simulink model "sampleModel1907"  (R2023a)
settings: Solver=VariableStepAuto  StartTime=0.0  StopTime=10.0  RelTol=1e-3
libraries: hdlsllib x5, simulink x4
settings Model: Creator=user1  LastModifiedBy=user1

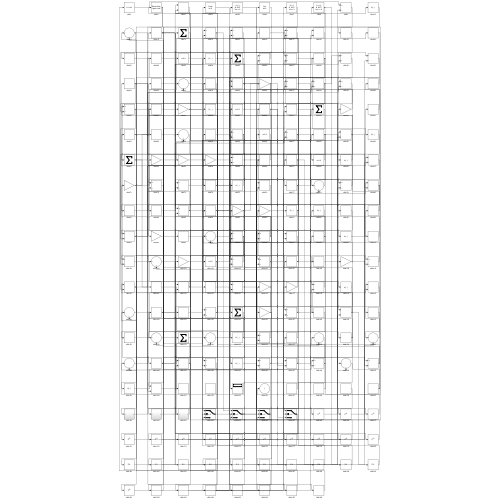
[thumbnail: Simulink's stored preview of the top-level diagram]
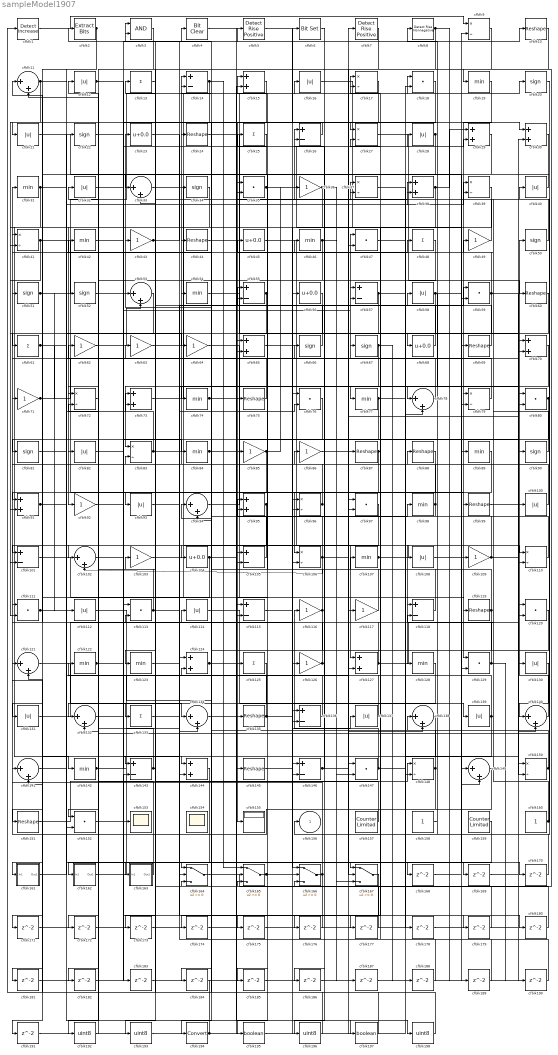
== system sampleModel1907 ==
  cfblk1 : simulink/Logic and Bit Operations/Detect Increase  vinit=0.0  OutDataTypeStr=boolean
      settings: LibrarySourceBlock=|
      | hdlsllib/Logic and Bit
      | Operations/Detect
      | Increase
  cfblk{10,24,44,60,69,75,87..88,99,119,135,145,151} (13 alike) : Reshape
  cfblk{12,16,21,28,32,40,58,82,93,100,108,112,114,130..131,137,139} (17 alike) : Abs  SaturateOnIntegerOverflow=off
  cfblk{14,26,55,57,101,105,115,118,136,143,146} (11 alike) : Sum  Inputs=+-
  cfblk{11,33,53,78,94,102,121,132,134,138,140..141,149} (13 alike) : Sum  Inputs=|++
  cfblk{36,43,49,62..64,71,85..86,92,103,109,116..117,126} (15 alike) : Gain
  cfblk{23,45,56,68,104} (5 alike) : Bias  Bias=0.0  SaturateOnIntegerOverflow=off
  cfblk{9,17,27,37,39,41,72,79,83,96,106,110,148,150} (14 alike) : Product  Inputs=*/  RndMeth=Zero  SaturateOnIntegerOverflow=on
  cfblk{19,31,42,46,54,74,77,84,89,98,107,122..123,128,142} (15 alike) : MinMax
  cfblk{18,35,47,59,76,80,97,111,113,120,129,147,152} (13 alike) : DotProduct  OutDataTypeStr=Inherit: Inherit via internal rule
  cfblk{15,29..30,38,65,70,73,91,95,124,127,144} (12 alike) : Sum
  cfblk{13,25,48,61,125,133} (6 alike) : Sum  Inputs=+
  cfblk153 : Scope
  cfblk154 : Scope
      settings: Floating=on
  cfblk155 : Display
  cfblk157 : hdlsllib/Sources/Counter Limited  uplimit=7  tsamp=-1
  cfblk158 : Constant  SampleTime=-1
  cfblk159 : hdlsllib/Sources/Counter Limited  uplimit=7  tsamp=-1
  cfblk160 : Constant  SampleTime=-1
  cfblk161 : Subsystem
      settings: LibrarySourceBlock=|
      | hdlsllib/Ports &
      | Subsystems/Subsystem
  cfblk162 : Subsystem
      settings: LibrarySourceBlock=|
      | hdlsllib/Ports &
      | Subsystems/Subsystem
  cfblk163 : Subsystem
      settings: LibrarySourceBlock=|
      | hdlsllib/Ports &
      | Subsystems/Subsystem
  cfblk{164..167} (4 alike) : Switch  SaturateOnIntegerOverflow=off  InputSameDT=off
  cfblk{168..191} (24 alike) : Delay  SampleTime=1
  cfblk{192..193,196,198} (4 alike) : DataTypeConversion  OutDataTypeStr=uint8  SaturateOnIntegerOverflow=off  RndMeth=Floor
  cfblk194 : DataTypeConversion  SaturateOnIntegerOverflow=off  RndMeth=Floor
  cfblk195 : DataTypeConversion  OutDataTypeStr=boolean  SaturateOnIntegerOverflow=off  RndMeth=Floor
  cfblk197 : DataTypeConversion  OutDataTypeStr=boolean  SaturateOnIntegerOverflow=off  RndMeth=Floor
  cfblk2 : simulink/Logic and Bit Operations/Extract Bits  bitsToExtract=Upper half  numBits=8  bitIdxRange=[0 7]  outScalingMode=Preserve fixed-point scaling
      settings: LibrarySourceBlock=|
      | hdlsllib/Logic and Bit
      | Operations/Extract Bits
  cfblk{20,22,34,50..52,66..67,81,90} (10 alike) : Signum
  cfblk3 : Logic  AllPortsSameDT=off  OutDataTypeStr=boolean
  cfblk4 : simulink/Logic and Bit Operations/Bit Clear  iBit=0
      settings: LibrarySourceBlock=|
      | hdlsllib/Logic and Bit
      | Operations/Bit Clear
  cfblk5 : hdlsllib/Logic and Bit Operations/Detect Rise Positive  vinit=0  OutDataTypeStr=boolean
  cfblk6 : simulink/Logic and Bit Operations/Bit Set  iBit=0
      settings: LibrarySourceBlock=|
      | hdlsllib/Logic and Bit
      | Operations/Bit Set
  cfblk7 : hdlsllib/Logic and Bit Operations/Detect Rise Positive  vinit=0  OutDataTypeStr=boolean
  cfblk8 : hdlsllib/Logic and Bit Operations/Detect Rise Nonnegative  vinit=0  OutDataTypeStr=boolean
  cfblk156 : Outport  VectorParamsAs1DForOutWhenUnconnected=off
  wires:
  cfblk18/1 -> cfblk155/1
  cfblk50/1 -> cfblk26/1
  cfblk66/1 -> cfblk13/1
  cfblk121/1 -> cfblk134/1
  cfblk140/1 -> cfblk50/1
  cfblk31/1 -> cfblk142/1, cfblk163/1(In1), cfblk197/1
  cfblk19/1 -> cfblk129/1
  cfblk34/1 -> cfblk92/1
  cfblk130/1 -> cfblk140/1
  cfblk112/1 -> cfblk144/1
  cfblk64/1 -> cfblk119/1
  cfblk61/1 -> cfblk112/1, cfblk38/2
  cfblk149/1 -> cfblk31/1
  cfblk51/1 -> cfblk16/1, cfblk39/2
  cfblk52/1 -> cfblk23/1
  cfblk84/1 -> cfblk99/1, cfblk58/1, cfblk37/2
  cfblk89/1 -> cfblk93/1
  cfblk45/1 -> cfblk79/1
  cfblk127/1 -> cfblk120/1, cfblk94/2
  cfblk87/1 -> cfblk106/1, cfblk37/1
  cfblk101/1 -> cfblk128/1
  cfblk143/1 -> cfblk111/1, cfblk173/1
  cfblk41/1 -> cfblk105/1, cfblk111/2
  cfblk114/1 -> cfblk139/1
  cfblk105/1 -> cfblk53/1
  cfblk98/1 -> cfblk14/1, cfblk95/2
  cfblk139/1 -> cfblk49/1, cfblk26/2, cfblk141/2
  cfblk20/1 -> cfblk156/1
  cfblk147/1 -> cfblk116/1, cfblk150/2
  cfblk74/1 -> cfblk127/1, cfblk14/2, cfblk110/2
  cfblk160/1 -> cfblk114/1, cfblk40/1
  cfblk72/1 -> cfblk102/1
  cfblk131/1 -> cfblk56/1
  cfblk103/1 -> cfblk149/1
  cfblk94/1 -> cfblk20/1
  cfblk26/1 -> cfblk21/1
  cfblk135/1 -> cfblk62/1, cfblk67/1
  cfblk44/1 -> cfblk68/1
  cfblk67/1 -> cfblk75/1, cfblk188/1
  cfblk136/1 -> cfblk12/1
  cfblk21/1 -> cfblk69/1
  cfblk53/1 -> cfblk131/1
  cfblk106/1 -> cfblk102/2, cfblk80/1, cfblk2/1
  cfblk33/1 -> cfblk166/1
  cfblk70/1 -> cfblk83/1
  cfblk77/1 -> cfblk82/1, cfblk80/2
  cfblk58/1 -> cfblk89/1, cfblk78/1, cfblk148/2
  cfblk79/1 -> cfblk51/1
  cfblk138/1 -> cfblk162/1(In1)
  cfblk40/1 -> cfblk33/1
  cfblk78/1 -> cfblk47/1
  cfblk73/1 -> cfblk18/1
  cfblk158/1 -> cfblk88/1
  cfblk91/1 -> cfblk73/1, cfblk48/1
  cfblk133/1 -> cfblk134/2
  cfblk62/1 -> cfblk53/2
  cfblk92/1 -> cfblk113/1
  cfblk83/1 -> cfblk106/2, cfblk73/2
  cfblk115/1 -> cfblk57/1
  cfblk157/1 -> cfblk103/1
  cfblk13/1 -> cfblk123/1
  cfblk95/1 -> cfblk121/2, cfblk193/1
  cfblk75/1 -> cfblk54/1
  cfblk150/1 -> cfblk138/1, cfblk72/2
  cfblk162/1(Out1) -> cfblk47/2
  cfblk57/1 -> cfblk145/1, cfblk78/2
  cfblk109/1 -> cfblk130/1, cfblk15/1
  cfblk148/1 -> cfblk44/1, cfblk177/1
  cfblk63/1 -> cfblk136/1
  cfblk71/1 -> cfblk70/1, cfblk52/1
  cfblk152/1 -> cfblk148/1
  cfblk119/1 -> cfblk107/1, cfblk185/1
  cfblk32/1 -> cfblk153/1
  cfblk86/1 -> cfblk87/1
  cfblk88/1 -> cfblk133/1
  cfblk17/1 -> cfblk74/1
  cfblk120/1 -> cfblk164/1
  cfblk65/1 -> cfblk118/1
  cfblk28/1 -> cfblk91/1, cfblk135/1
  cfblk80/1 -> cfblk115/1, cfblk171/1
  cfblk113/1 -> cfblk59/1, cfblk11/2
  cfblk25/1 -> cfblk115/2
  cfblk107/1 -> cfblk110/1, cfblk27/2
  cfblk12/1 -> cfblk84/1, cfblk152/1, cfblk179/1, cfblk180/1
  cfblk46/1 -> cfblk147/2, cfblk167/3, cfblk172/1
  cfblk116/1 -> cfblk95/1, cfblk165/2
  cfblk146/1 -> cfblk46/1, cfblk138/2
  cfblk142/1 -> cfblk76/2, cfblk29/2
  cfblk29/1 -> cfblk125/1
  cfblk43/1 -> cfblk10/1, cfblk176/1
  cfblk99/1 -> cfblk90/1
  cfblk35/1 -> cfblk109/1, cfblk28/1
  cfblk85/1 -> cfblk161/1(In1), cfblk36/1
  cfblk8/1 -> cfblk33/2, cfblk189/1
  cfblk164/1 -> cfblk19/1
  cfblk110/1 -> cfblk41/1
  cfblk47/1 -> cfblk108/1
  cfblk36/1 -> cfblk91/2, cfblk61/1, cfblk187/1
  cfblk24/1 -> cfblk126/1
  cfblk100/1 -> cfblk17/1
  cfblk55/1 -> cfblk132/1, cfblk184/1
  cfblk82/1 -> cfblk24/1
  cfblk118/1 -> cfblk34/1
  cfblk15/1 -> cfblk104/1
  cfblk151/1 -> cfblk117/1
  cfblk124/1 -> cfblk98/1, cfblk94/1
  cfblk48/1 -> cfblk146/2
  cfblk23/1 -> cfblk77/1
  cfblk90/1 -> cfblk39/1
  cfblk111/1 -> cfblk63/1, cfblk181/1
  cfblk16/1 -> cfblk149/2
  cfblk39/1 -> cfblk167/1
  cfblk5/1 -> cfblk27/1
  cfblk1/1 -> cfblk9/1
  cfblk68/1 -> cfblk43/1
  cfblk159/1 -> cfblk194/1
  cfblk54/1 -> cfblk150/1
  cfblk2/1 -> cfblk101/1, cfblk152/2
  cfblk166/1 -> cfblk141/1, cfblk165/3
  cfblk76/1 -> cfblk96/2
  cfblk42/1 -> cfblk5/1
  cfblk9/1 -> cfblk65/2
  cfblk125/1 -> cfblk132/2
  cfblk96/1 -> cfblk71/1, cfblk3/2
  cfblk104/1 -> cfblk85/1, cfblk151/1
  cfblk27/1 -> cfblk60/1
  cfblk30/1 -> cfblk35/2
  cfblk137/1 -> cfblk122/1
  cfblk161/1(Out1) -> cfblk66/1
  cfblk117/1 -> cfblk86/1
  cfblk56/1 -> cfblk143/1
  cfblk129/1 -> cfblk8/1, cfblk190/1
  cfblk122/1 -> cfblk57/2, cfblk144/2
  cfblk141/1 -> cfblk124/2
  cfblk123/1 -> cfblk55/1
  cfblk163/1(Out1) -> cfblk42/1
  cfblk81/1 -> cfblk22/1
  cfblk49/1 -> cfblk3/1
  cfblk38/1 -> cfblk136/2, cfblk29/1, cfblk55/2
  cfblk10/1 -> cfblk167/2
  cfblk3/1 -> cfblk72/1
  cfblk165/1 -> cfblk137/1, cfblk38/1
  cfblk14/1 -> cfblk81/1, cfblk165/1
  cfblk22/1 -> cfblk30/1
  cfblk69/1 -> cfblk45/1
  cfblk60/1 -> cfblk101/2
  cfblk126/1 -> cfblk11/1, cfblk186/1
  cfblk59/1 -> cfblk100/1, cfblk97/2, cfblk25/1
  cfblk11/1 -> cfblk64/1, cfblk41/2
  cfblk134/1 -> cfblk105/2
  cfblk102/1 -> cfblk168/1
  cfblk168/1 -> cfblk59/2
  cfblk145/1 -> cfblk169/1
  cfblk169/1 -> cfblk140/2
  cfblk108/1 -> cfblk170/1
  cfblk170/1 -> cfblk118/2
  cfblk171/1 -> cfblk120/2
  cfblk172/1 -> cfblk76/1
  cfblk173/1 -> cfblk129/2
  cfblk167/1 -> cfblk174/1
  cfblk174/1 -> cfblk96/1
  cfblk93/1 -> cfblk175/1
  cfblk175/1 -> cfblk147/1
  cfblk176/1 -> cfblk164/2
  cfblk177/1 -> cfblk166/2
  cfblk37/1 -> cfblk178/1
  cfblk178/1 -> cfblk70/2
  cfblk179/1 -> cfblk83/2
  cfblk180/1 -> cfblk166/3
  cfblk181/1 -> cfblk143/2
  cfblk144/1 -> cfblk182/1
  cfblk182/1 -> cfblk35/1
  cfblk132/1 -> cfblk183/1
  cfblk183/1 -> cfblk127/2
  cfblk184/1 -> cfblk1/1
  cfblk185/1 -> cfblk79/2
  cfblk186/1 -> cfblk30/2
  cfblk187/1 -> cfblk9/2
  cfblk188/1 -> cfblk124/1
  cfblk189/1 -> cfblk17/2
  cfblk190/1 -> cfblk164/3
  cfblk97/1 -> cfblk191/1
  cfblk191/1 -> cfblk65/1
  cfblk7/1 -> cfblk192/1
  cfblk192/1 -> cfblk32/1
  cfblk193/1 -> cfblk7/1
  cfblk194/1 -> cfblk15/2, cfblk113/2, cfblk18/2, cfblk97/1
  cfblk128/1 -> cfblk195/1
  cfblk195/1 -> cfblk6/1
  cfblk6/1 -> cfblk196/1
  cfblk196/1 -> cfblk146/1
  cfblk197/1 -> cfblk4/1
  cfblk4/1 -> cfblk198/1
  cfblk198/1 -> cfblk121/1

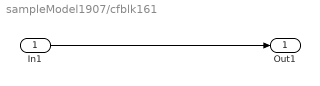
== system sampleModel1907/cfblk161 ==
  In1 : Inport
  Out1 : Outport
  wires:
  In1/1 -> Out1/1

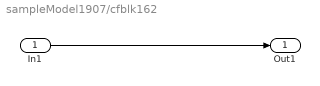
== system sampleModel1907/cfblk162 ==
  In1 : Inport
  Out1 : Outport
  wires:
  In1/1 -> Out1/1

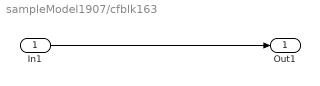
== system sampleModel1907/cfblk163 ==
  In1 : Inport
  Out1 : Outport
  wires:
  In1/1 -> Out1/1
